simulink model "non_linear_model"  (R2018b)
settings: Solver=VariableStepAuto  StartTime=0.0  StopTime=10  RelTol=1e-3
values from neighbouring files (symbols this model uses):
  b = 1.5    [dettagli_auto.mat]
  ca = 1500    [dettagli_auto.mat]
  cp = 1600    [dettagli_auto.mat]
  g = 9.8    [dettagli_auto.mat]
  I = 24225    [dettagli_auto.mat]
  ka = 50000    [dettagli_auto.mat]
  Khinf = c2d(Khinf,Ts,'tustin')    [controllore_hinf.m]
  kp = 48000    [dettagli_auto.mat]
  lk = 1.125    [dettagli_auto.mat]
  m = 1600    [dettagli_auto.mat]
  noise_x = 0.0025    [dettagli_auto.mat]
  Ts = 0.01    [dettagli_auto.mat]
  x0 = [1.125 0 0 0]    [dettagli_auto.mat]
undefined symbols (not defined in the file or in its folder): int_lqg, int_pp, obs_lqg, obs_pp, sigbuilder_block
settings Model: Creator=cirom  LastModifiedBy=cirom

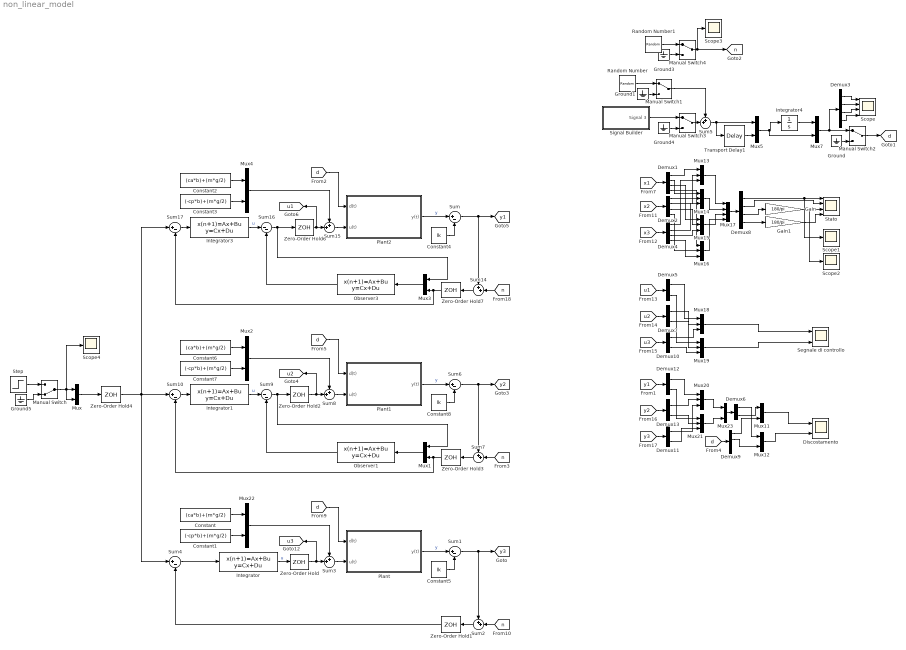
== system non_linear_model ==
  Constant : Constant  Value=(ca*b)+(m*g/2)
  Constant1 : Constant  Value=(-cp*b)+(m*g/2)
  Constant2 : Constant  Value=(ca*b)+(m*g/2)
  Constant3 : Constant  Value=(-cp*b)+(m*g/2)
  Constant4 : Constant  Value=lk
  Constant5 : Constant  Value=lk
  Constant6 : Constant  Value=(ca*b)+(m*g/2)
  Constant7 : Constant  Value=(-cp*b)+(m*g/2)
  Constant8 : Constant  Value=lk
  Demux{1..4,8..9} (6 alike) : Demux
  Demux{5..7,10..13} (7 alike) : Demux  Outputs=2
  Discostamento : Scope  NumInputPorts=2
  Gain : Gain  Gain=180/pi
  Gain1 : Gain  Gain=180/pi
  Ground{,1,3..5} (5 alike) : Ground
  Integrator : DiscreteStateSpace  A=Khinf.A  B=Khinf.B  C=Khinf.C  D=Khinf.D  SampleTime=-1
  Integrator1 : DiscreteStateSpace  A=int_lqg.A  B=int_lqg.B  C=int_lqg.C  D=int_lqg.D  SampleTime=-1
  Integrator3 : DiscreteStateSpace  A=int_pp.A  B=int_pp.B  C=int_pp.C  D=int_pp.D  SampleTime=-1
  Integrator4 : Integrator
  Manual Switch : ManualSwitch  CurrentSetting=0
  Manual Switch{1..4} (4 alike) : ManualSwitch
  Mux{,1..5,7,11..12,22..23} (11 alike) : Mux  Inputs=2
  Mux{13..16,18..21} (8 alike) : Mux  Inputs=3
  Mux17 : Mux
  Observer1 : DiscreteStateSpace  A=obs_lqg.A  B=obs_lqg.B  C=obs_lqg.C  D=obs_lqg.D  SampleTime=-1
  Observer3 : DiscreteStateSpace  A=obs_pp.A  B=obs_pp.B  C=obs_pp.C  D=obs_pp.D  SampleTime=-1
  Plant : Subsystem
  Plant1 : Subsystem
  Plant2 : Subsystem
  Random Number : RandomNumber  Variance=noise_x  SampleTime=0.01
  Random Number1 : RandomNumber  Variance=[1, 1] * 10^-4  SampleTime=0.001
  Scope : Scope  NumInputPorts=4
  Scope{1..4} (4 alike) : Scope
  Segnale di controllo : Scope  NumInputPorts=2
  Signal Builder : Subsystem  Tag=STV Subsys  LoadFcn=sigbuilder_block('load');  StartFcn=sigbuilder_block('start');  StopFcn=sigbuilder_block('stop');  ClipboardFcn=sigbuilder_block('clipboard');  mask(Sigbuilder block){tuvar=[0:10]}
      mask help: Simulink:masks:SigbuilderBlock_MD
      mask init:
      | if ~strcmp(get_param(bdroot(gcbh),'SimulationStatus'),'stopped') tuvar = sigbuilder_block('maskInit'); end
      settings: CopyFcn=sigbuilder_block('copy');  DeleteFcn=sigbuilder_block('delete');  ModelCloseFcn=sigbuilder_block('modelClose');  PreSaveFcn=sigbuilder_block('preSave');  PauseFcn=sigbuilder_block('pause');  ContinueFcn=sigbuilder_block('continue');  NameChangeFcn=sigbuilder_block('namechange');  OpenFcn=sigbuilder_block('open',[6 22.5 1012.5 455.25 ]);  CloseFcn=sigbuilder_block('close');
      mask Display: plot(0, 0, 100, 100,[2, 2, 32, 32, 2], [68, 8, 8, 68, 68],[32, 2], [38, 38], [32, 19, 2],[53, 60, 44], [32, 17, 17, 2],[16, 16, 31, 31]);txt = getActiveGroup(gcbh);text(2, 100, txt,'verticalAlignment', 'top');
  Stato : Scope  NumInputPorts=4
  Step : Step  After=0.05  SampleTime=0
  Sum{,1,4,6,10,17} (6 alike) : Sum  Inputs=|+-
  Sum{2..3,5,7..8,14..15} (7 alike) : Sum  Inputs=++|
  Sum16 : Sum  Inputs=|--
  Sum9 : Sum  Inputs=|--
  Transport Delay1 : TransportDelay  DelayTime=0.4
  Zero-Order Hold{,1..4,6..7} (7 alike) : ZeroOrderHold  SampleTime=Ts
  tag scope: d=global, n=global, u1=global, u2=global, u3=global, y1=global, y2=global, y3=global
  wires:
  Mux11/1 -> Discostamento/1
  [d] -> Demux9/1
  Mux17/1 -> Demux8/1
  Demux9/1 -> Mux11/2
  Demux9/2 -> Mux12/2
  Demux8/2 -> Stato/2
  Demux8/4 -> Gain1/1
  Gain1/1 -> Stato/4
  Demux8/1 -> Scope1/1, Stato/1
  Demux8/3 -> Gain/1
  Gain/1 -> Scope2/1, Stato/3
  Mux18/1 -> Segnale di controllo/1
  Mux19/1 -> Segnale di controllo/2
  [x2] -> Demux2/1
  [x3] -> Demux4/1
  Mux13/1 -> Mux17/1
  Mux14/1 -> Mux17/2
  Mux15/1 -> Mux17/3
  Mux16/1 -> Mux17/4
  Demux1/1 -> Mux13/1
  Demux2/1 -> Mux13/2
  Demux4/1 -> Mux13/3
  Demux1/2 -> Mux14/1
  Demux2/2 -> Mux14/2
  Demux4/2 -> Mux14/3
  Demux1/3 -> Mux15/1
  Demux2/3 -> Mux15/2
  Demux4/3 -> Mux15/3
  Demux1/4 -> Mux16/1
  Demux2/4 -> Mux16/2
  Demux4/4 -> Mux16/3
  Demux5/1 -> Mux18/1
  Demux5/2 -> Mux19/1
  Demux7/1 -> Mux18/2
  Demux7/2 -> Mux19/2
  Demux10/1 -> Mux18/3
  Demux10/2 -> Mux19/3
  [u2] -> Demux7/1
  [u3] -> Demux10/1
  Demux11/2 -> Mux21/3
  Demux12/2 -> Mux21/1
  Demux12/1 -> Mux20/1
  Mux20/1 -> Mux23/1
  Demux13/2 -> Mux21/2
  Mux23/1 -> Demux6/1
  Demux13/1 -> Mux20/2
  Demux11/1 -> Mux20/3
  Mux21/1 -> Mux23/2
  [y2] -> Demux13/1
  [y3] -> Demux11/1
  Manual Switch4/1 -> Scope3/1, [n]
  Ground3/1 -> Manual Switch4/2
  Random Number1/1 -> Manual Switch4/1
  Demux6/1 -> Mux12/1
  Demux6/2 -> Mux11/1
  Integrator3/1 -> Sum16/1  "u"
  [d] -> Plant2/1(d(t))
  Plant2/1(y(t)) -> Sum/1  "y"
  Sum17/1 -> Integrator3/1
  Mux3/1 -> Observer3/1
  Constant2/1 -> Mux4/1
  Observer3/1 -> Sum16/2
  Sum15/1 -> Plant2/2(u(t))
  Mux4/1 -> Sum15/1
  [n] -> Sum14/2
  Constant3/1 -> Mux4/2
  Zero-Order Hold7/1 -> Sum17/2, Mux3/2
  Sum16/1 -> Mux3/1, Zero-Order Hold6/1
  Sum14/1 -> Zero-Order Hold7/1
  Sum/1 -> Sum14/1, [y1]
  Zero-Order Hold6/1 -> [u1], Sum15/2
  Constant4/1 -> Sum/2
  Demux3/4 -> Scope/4
  Demux3/3 -> Scope/3
  Random Number/1 -> Manual Switch1/1
  Ground4/1 -> Manual Switch3/2
  Demux3/2 -> Scope/2
  Mux7/1 -> Demux3/1, Manual Switch2/1
  Manual Switch3/1 -> Sum5/2
  Ground/1 -> Manual Switch2/2
  Ground1/1 -> Manual Switch1/2
  Manual Switch1/1 -> Sum5/1
  Sum5/1 -> Transport Delay1/1, Mux5/1
  Manual Switch2/1 -> [d]
  Mux5/1 -> Mux7/2, Integrator4/1
  Transport Delay1/1 -> Mux5/2
  Demux3/1 -> Scope/1
  Integrator4/1 -> Mux7/1
  Signal Builder/1(Signal 3) -> Manual Switch3/1
  [x1] -> Demux1/1
  [u1] -> Demux5/1
  [y1] -> Demux12/1
  Sum3/1 -> Plant/2(u(t))
  Zero-Order Hold/1 -> Sum3/2, [u3]
  [n] -> Sum2/2
  Plant/1(y(t)) -> Sum1/1  "y"
  Constant5/1 -> Sum1/2
  Sum2/1 -> Zero-Order Hold1/1
  Integrator/1 -> Zero-Order Hold/1  "u"
  [d] -> Plant/1(d(t))
  Mux22/1 -> Sum3/1
  Zero-Order Hold4/1 -> Sum4/1, Sum17/1, Sum10/1
  Constant1/1 -> Mux22/2
  Sum1/1 -> Sum2/1, [y3]
  Zero-Order Hold1/1 -> Sum4/2
  Sum4/1 -> Integrator/1
  Constant/1 -> Mux22/1
  Mux12/1 -> Discostamento/2
  [n] -> Sum7/2
  Zero-Order Hold2/1 -> [u2], Sum8/2
  Sum9/1 -> Mux1/1, Zero-Order Hold2/1
  Mux1/1 -> Observer1/1
  Observer1/1 -> Sum9/2
  Sum6/1 -> Sum7/1, [y2]
  Sum7/1 -> Zero-Order Hold3/1
  Integrator1/1 -> Sum9/1  "u"
  Constant7/1 -> Mux2/2
  Mux2/1 -> Sum8/1
  Sum8/1 -> Plant1/2(u(t))
  Sum10/1 -> Integrator1/1
  Plant1/1(y(t)) -> Sum6/1  "y"
  [d] -> Plant1/1(d(t))
  Constant6/1 -> Mux2/1
  Zero-Order Hold3/1 -> Sum10/2, Mux1/2
  Constant8/1 -> Sum6/2
  Step/1 -> Manual Switch/1
  Ground5/1 -> Manual Switch/2
  Manual Switch/1 -> Scope4/1, Mux/2, Mux/1
  Mux/1 -> Zero-Order Hold4/1

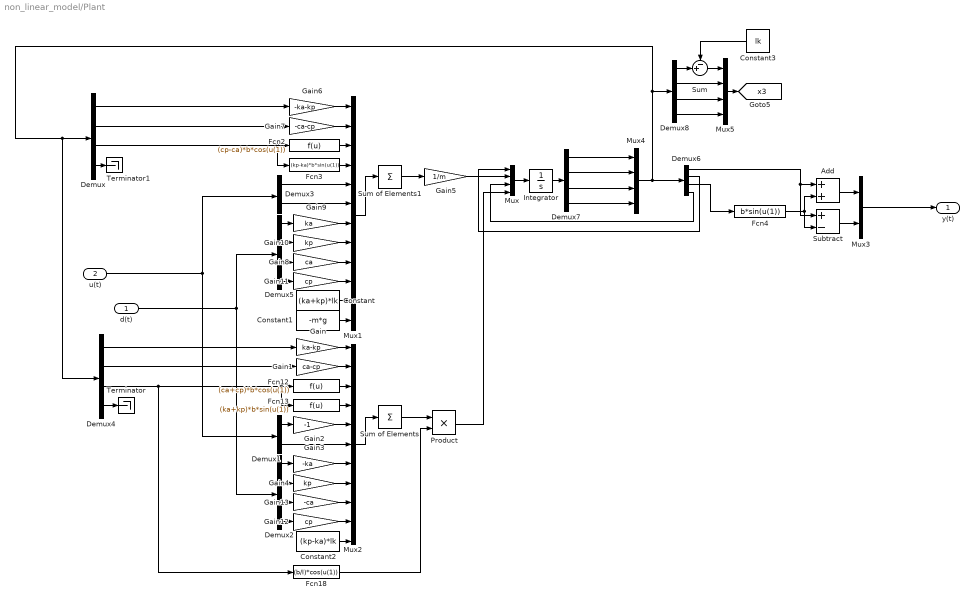
== system non_linear_model/Plant ==
  d(t) : Inport
  u(t) : Inport  Port=2
  Add : Sum
  Constant : Constant  Value=(ka+kp)*lk
  Constant1 : Constant  Value=-m*g
  Constant2 : Constant  Value=(kp-ka)*lk
  Constant3 : Constant  Value=lk
  Demux{,2,4..8} (7 alike) : Demux
  Demux1 : Demux  Outputs=2
  Demux3 : Demux  Outputs=2
  Fcn12 : Fcn  Expr=(ca+cp)*b*cos(u(1))
  Fcn13 : Fcn  Expr=(ka+kp)*b*sin(u(1))
  Fcn18 : Fcn  Expr=(b/I)*cos(u(1))
  Fcn2 : Fcn  Expr=(cp-ca)*b*cos(u(1))
  Fcn3 : Fcn  Expr=(kp-ka)*b*sin(u(1))
  Fcn4 : Fcn  Expr=b*sin(u(1))
  Gain : Gain  Gain=ka-kp
  Gain1 : Gain  Gain=ca-cp
  Gain10 : Gain  Gain=kp
  Gain11 : Gain  Gain=cp
  Gain12 : Gain  Gain=cp
  Gain13 : Gain  Gain=-ca
  Gain2 : Gain  Gain=-1
  Gain3 : Gain  Gain=-ka
  Gain4 : Gain  Gain=kp
  Gain5 : Gain  Gain=1/m
  Gain6 : Gain  Gain=-ka-kp
  Gain7 : Gain  Gain=-ca-cp
  Gain8 : Gain  Gain=ca
  Gain9 : Gain  Gain=ka
  Integrator : Integrator  InitialCondition=x0
  Mux : Mux
  Mux1 : Mux  Inputs=12
  Mux2 : Mux  Inputs=11
  Mux3 : Mux  Inputs=2
  Mux4 : Mux
  Mux5 : Mux
  Product : Product
  Subtract : Sum  Inputs=+-
  Sum : Sum  Inputs=-+|
  Sum of Elements : Sum  Inputs=+
  Sum of Elements1 : Sum  Inputs=+
  Terminator : Terminator
  Terminator1 : Terminator
  y(t) : Outport
  tag scope: x3=global
  wires:
  Mux/1 -> Integrator/1
  u(t)/1 -> Demux3/1, Demux1/1
  Mux1/1 -> Sum of Elements1/1
  Demux2/1 -> Gain3/1
  Demux2/2 -> Gain4/1
  Gain3/1 -> Mux2/7
  Gain4/1 -> Mux2/8
  Gain/1 -> Mux2/1
  Gain1/1 -> Mux2/2
  Fcn12/1 -> Mux2/3
  Mux2/1 -> Sum of Elements/1
  Fcn13/1 -> Mux2/4
  Sum of Elements/1 -> Product/1
  Fcn18/1 -> Product/2
  Gain2/1 -> Mux2/5
  Product/1 -> Mux/4
  Sum of Elements1/1 -> Gain5/1
  Gain5/1 -> Mux/2
  Gain9/1 -> Mux1/7
  Demux3/1 -> Mux1/5
  Fcn2/1 -> Mux1/3
  Gain10/1 -> Mux1/8
  Fcn3/1 -> Mux1/4
  Gain7/1 -> Mux1/2
  Gain6/1 -> Mux1/1
  Demux3/2 -> Mux1/6
  Demux1/1 -> Gain2/1
  Demux1/2 -> Mux2/6
  d(t)/1 -> Demux2/1, Demux5/1
  Demux/1 -> Gain6/1
  Demux/2 -> Gain7/1
  Demux/3 -> Fcn3/1, Fcn2/1
  Demux4/1 -> Gain/1
  Demux4/2 -> Gain1/1
  Demux4/3 -> Fcn18/1, Fcn13/1, Fcn12/1
  Demux4/4 -> Terminator/1
  Demux5/1 -> Gain9/1
  Demux5/2 -> Gain10/1
  Demux/4 -> Terminator1/1
  Demux6/2 -> Mux/1
  Demux6/4 -> Mux/3
  Demux6/1 -> Subtract/1, Add/1
  Fcn4/1 -> Add/2, Subtract/2
  Add/1 -> Mux3/1
  Subtract/1 -> Mux3/2
  Mux3/1 -> y(t)/1
  Demux6/3 -> Fcn4/1
  Mux4/1 -> Demux8/1, Demux4/1, Demux/1, Demux6/1
  Integrator/1 -> Demux7/1
  Demux7/1 -> Mux4/1
  Demux7/2 -> Mux4/2
  Demux7/3 -> Mux4/3
  Demux7/4 -> Mux4/4
  Demux5/3 -> Gain8/1
  Demux5/4 -> Gain11/1
  Gain8/1 -> Mux1/9
  Gain11/1 -> Mux1/10
  Demux2/3 -> Gain13/1
  Demux2/4 -> Gain12/1
  Gain13/1 -> Mux2/9
  Gain12/1 -> Mux2/10
  Constant/1 -> Mux1/11
  Constant1/1 -> Mux1/12
  Constant2/1 -> Mux2/11
  Sum/1 -> Mux5/1
  Demux8/1 -> Sum/2
  Demux8/2 -> Mux5/2
  Demux8/3 -> Mux5/3
  Demux8/4 -> Mux5/4
  Mux5/1 -> [x3]
  Constant3/1 -> Sum/1

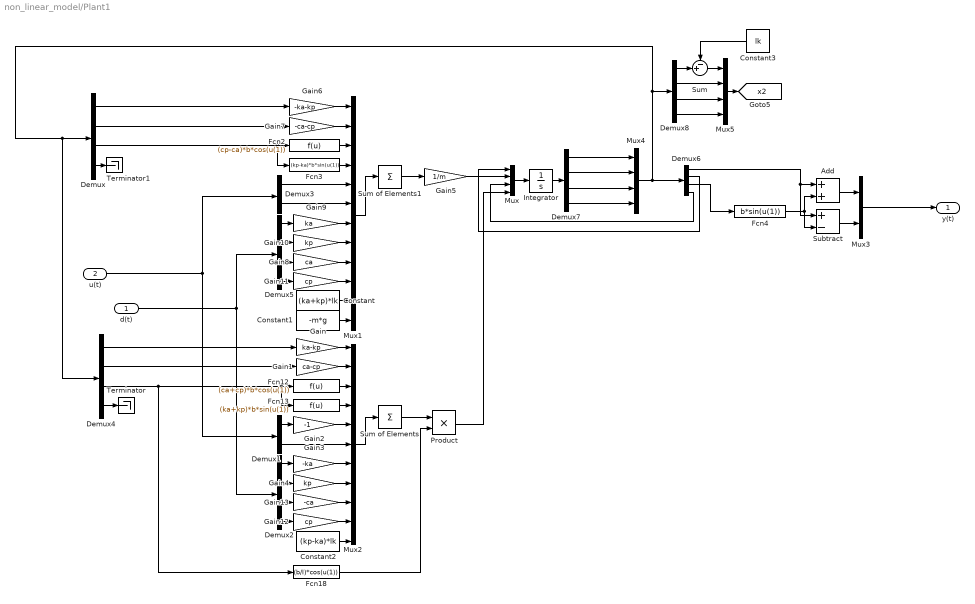
== system non_linear_model/Plant1 ==
  d(t) : Inport
  u(t) : Inport  Port=2
  Add : Sum
  Constant : Constant  Value=(ka+kp)*lk
  Constant1 : Constant  Value=-m*g
  Constant2 : Constant  Value=(kp-ka)*lk
  Constant3 : Constant  Value=lk
  Demux{,2,4..8} (7 alike) : Demux
  Demux1 : Demux  Outputs=2
  Demux3 : Demux  Outputs=2
  Fcn12 : Fcn  Expr=(ca+cp)*b*cos(u(1))
  Fcn13 : Fcn  Expr=(ka+kp)*b*sin(u(1))
  Fcn18 : Fcn  Expr=(b/I)*cos(u(1))
  Fcn2 : Fcn  Expr=(cp-ca)*b*cos(u(1))
  Fcn3 : Fcn  Expr=(kp-ka)*b*sin(u(1))
  Fcn4 : Fcn  Expr=b*sin(u(1))
  Gain : Gain  Gain=ka-kp
  Gain1 : Gain  Gain=ca-cp
  Gain10 : Gain  Gain=kp
  Gain11 : Gain  Gain=cp
  Gain12 : Gain  Gain=cp
  Gain13 : Gain  Gain=-ca
  Gain2 : Gain  Gain=-1
  Gain3 : Gain  Gain=-ka
  Gain4 : Gain  Gain=kp
  Gain5 : Gain  Gain=1/m
  Gain6 : Gain  Gain=-ka-kp
  Gain7 : Gain  Gain=-ca-cp
  Gain8 : Gain  Gain=ca
  Gain9 : Gain  Gain=ka
  Integrator : Integrator  InitialCondition=x0
  Mux : Mux
  Mux1 : Mux  Inputs=12
  Mux2 : Mux  Inputs=11
  Mux3 : Mux  Inputs=2
  Mux4 : Mux
  Mux5 : Mux
  Product : Product
  Subtract : Sum  Inputs=+-
  Sum : Sum  Inputs=-+|
  Sum of Elements : Sum  Inputs=+
  Sum of Elements1 : Sum  Inputs=+
  Terminator : Terminator
  Terminator1 : Terminator
  y(t) : Outport
  tag scope: x2=global
  wires:
  Mux/1 -> Integrator/1
  u(t)/1 -> Demux3/1, Demux1/1
  Mux1/1 -> Sum of Elements1/1
  Demux2/1 -> Gain3/1
  Demux2/2 -> Gain4/1
  Gain3/1 -> Mux2/7
  Gain4/1 -> Mux2/8
  Gain/1 -> Mux2/1
  Gain1/1 -> Mux2/2
  Fcn12/1 -> Mux2/3
  Mux2/1 -> Sum of Elements/1
  Fcn13/1 -> Mux2/4
  Sum of Elements/1 -> Product/1
  Fcn18/1 -> Product/2
  Gain2/1 -> Mux2/5
  Product/1 -> Mux/4
  Sum of Elements1/1 -> Gain5/1
  Gain5/1 -> Mux/2
  Gain9/1 -> Mux1/7
  Demux3/1 -> Mux1/5
  Fcn2/1 -> Mux1/3
  Gain10/1 -> Mux1/8
  Fcn3/1 -> Mux1/4
  Gain7/1 -> Mux1/2
  Gain6/1 -> Mux1/1
  Demux3/2 -> Mux1/6
  Demux1/1 -> Gain2/1
  Demux1/2 -> Mux2/6
  d(t)/1 -> Demux2/1, Demux5/1
  Demux/1 -> Gain6/1
  Demux/2 -> Gain7/1
  Demux/3 -> Fcn3/1, Fcn2/1
  Demux4/1 -> Gain/1
  Demux4/2 -> Gain1/1
  Demux4/3 -> Fcn18/1, Fcn13/1, Fcn12/1
  Demux4/4 -> Terminator/1
  Demux5/1 -> Gain9/1
  Demux5/2 -> Gain10/1
  Demux/4 -> Terminator1/1
  Demux6/2 -> Mux/1
  Demux6/4 -> Mux/3
  Demux6/1 -> Subtract/1, Add/1
  Fcn4/1 -> Add/2, Subtract/2
  Add/1 -> Mux3/1
  Subtract/1 -> Mux3/2
  Mux3/1 -> y(t)/1
  Demux6/3 -> Fcn4/1
  Mux4/1 -> Demux8/1, Demux4/1, Demux/1, Demux6/1
  Integrator/1 -> Demux7/1
  Demux7/1 -> Mux4/1
  Demux7/2 -> Mux4/2
  Demux7/3 -> Mux4/3
  Demux7/4 -> Mux4/4
  Demux5/3 -> Gain8/1
  Demux5/4 -> Gain11/1
  Gain8/1 -> Mux1/9
  Gain11/1 -> Mux1/10
  Demux2/3 -> Gain13/1
  Demux2/4 -> Gain12/1
  Gain13/1 -> Mux2/9
  Gain12/1 -> Mux2/10
  Constant/1 -> Mux1/11
  Constant1/1 -> Mux1/12
  Constant2/1 -> Mux2/11
  Sum/1 -> Mux5/1
  Demux8/1 -> Sum/2
  Demux8/2 -> Mux5/2
  Demux8/3 -> Mux5/3
  Demux8/4 -> Mux5/4
  Mux5/1 -> [x2]
  Constant3/1 -> Sum/1

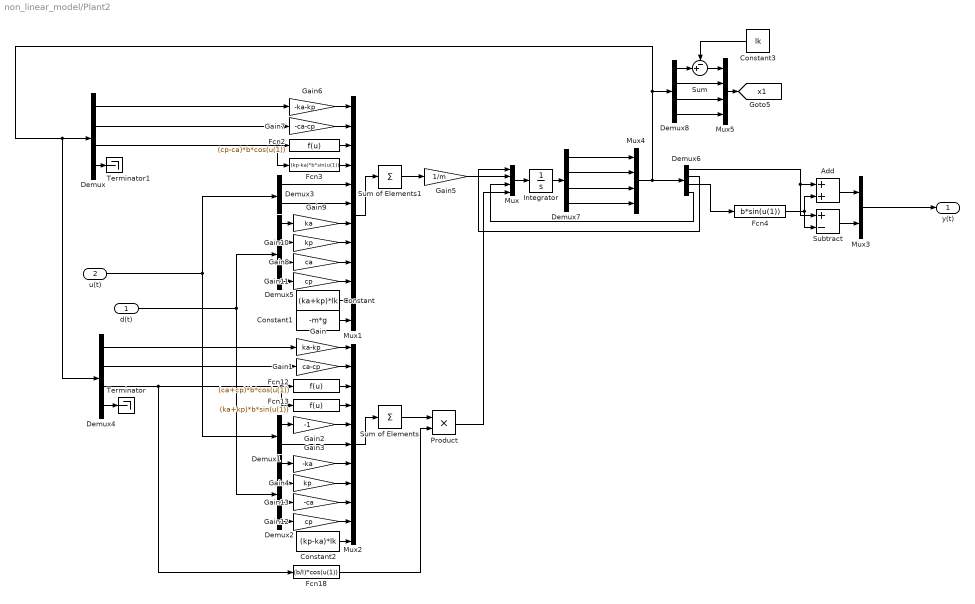
== system non_linear_model/Plant2 ==
  d(t) : Inport
  u(t) : Inport  Port=2
  Add : Sum
  Constant : Constant  Value=(ka+kp)*lk
  Constant1 : Constant  Value=-m*g
  Constant2 : Constant  Value=(kp-ka)*lk
  Constant3 : Constant  Value=lk
  Demux{,2,4..8} (7 alike) : Demux
  Demux1 : Demux  Outputs=2
  Demux3 : Demux  Outputs=2
  Fcn12 : Fcn  Expr=(ca+cp)*b*cos(u(1))
  Fcn13 : Fcn  Expr=(ka+kp)*b*sin(u(1))
  Fcn18 : Fcn  Expr=(b/I)*cos(u(1))
  Fcn2 : Fcn  Expr=(cp-ca)*b*cos(u(1))
  Fcn3 : Fcn  Expr=(kp-ka)*b*sin(u(1))
  Fcn4 : Fcn  Expr=b*sin(u(1))
  Gain : Gain  Gain=ka-kp
  Gain1 : Gain  Gain=ca-cp
  Gain10 : Gain  Gain=kp
  Gain11 : Gain  Gain=cp
  Gain12 : Gain  Gain=cp
  Gain13 : Gain  Gain=-ca
  Gain2 : Gain  Gain=-1
  Gain3 : Gain  Gain=-ka
  Gain4 : Gain  Gain=kp
  Gain5 : Gain  Gain=1/m
  Gain6 : Gain  Gain=-ka-kp
  Gain7 : Gain  Gain=-ca-cp
  Gain8 : Gain  Gain=ca
  Gain9 : Gain  Gain=ka
  Integrator : Integrator  InitialCondition=x0
  Mux : Mux
  Mux1 : Mux  Inputs=12
  Mux2 : Mux  Inputs=11
  Mux3 : Mux  Inputs=2
  Mux4 : Mux
  Mux5 : Mux
  Product : Product
  Subtract : Sum  Inputs=+-
  Sum : Sum  Inputs=-+|
  Sum of Elements : Sum  Inputs=+
  Sum of Elements1 : Sum  Inputs=+
  Terminator : Terminator
  Terminator1 : Terminator
  y(t) : Outport
  tag scope: x1=global
  wires:
  Mux/1 -> Integrator/1
  u(t)/1 -> Demux3/1, Demux1/1
  Mux1/1 -> Sum of Elements1/1
  Demux2/1 -> Gain3/1
  Demux2/2 -> Gain4/1
  Gain3/1 -> Mux2/7
  Gain4/1 -> Mux2/8
  Gain/1 -> Mux2/1
  Gain1/1 -> Mux2/2
  Fcn12/1 -> Mux2/3
  Mux2/1 -> Sum of Elements/1
  Fcn13/1 -> Mux2/4
  Sum of Elements/1 -> Product/1
  Fcn18/1 -> Product/2
  Gain2/1 -> Mux2/5
  Product/1 -> Mux/4
  Sum of Elements1/1 -> Gain5/1
  Gain5/1 -> Mux/2
  Gain9/1 -> Mux1/7
  Demux3/1 -> Mux1/5
  Fcn2/1 -> Mux1/3
  Gain10/1 -> Mux1/8
  Fcn3/1 -> Mux1/4
  Gain7/1 -> Mux1/2
  Gain6/1 -> Mux1/1
  Demux3/2 -> Mux1/6
  Demux1/1 -> Gain2/1
  Demux1/2 -> Mux2/6
  d(t)/1 -> Demux2/1, Demux5/1
  Demux/1 -> Gain6/1
  Demux/2 -> Gain7/1
  Demux/3 -> Fcn3/1, Fcn2/1
  Demux4/1 -> Gain/1
  Demux4/2 -> Gain1/1
  Demux4/3 -> Fcn18/1, Fcn13/1, Fcn12/1
  Demux4/4 -> Terminator/1
  Demux5/1 -> Gain9/1
  Demux5/2 -> Gain10/1
  Demux/4 -> Terminator1/1
  Demux6/2 -> Mux/1
  Demux6/4 -> Mux/3
  Demux6/1 -> Subtract/1, Add/1
  Fcn4/1 -> Add/2, Subtract/2
  Add/1 -> Mux3/1
  Subtract/1 -> Mux3/2
  Mux3/1 -> y(t)/1
  Demux6/3 -> Fcn4/1
  Mux4/1 -> Demux8/1, Demux4/1, Demux/1, Demux6/1
  Integrator/1 -> Demux7/1
  Demux7/1 -> Mux4/1
  Demux7/2 -> Mux4/2
  Demux7/3 -> Mux4/3
  Demux7/4 -> Mux4/4
  Demux5/3 -> Gain8/1
  Demux5/4 -> Gain11/1
  Gain8/1 -> Mux1/9
  Gain11/1 -> Mux1/10
  Demux2/3 -> Gain13/1
  Demux2/4 -> Gain12/1
  Gain13/1 -> Mux2/9
  Gain12/1 -> Mux2/10
  Constant/1 -> Mux1/11
  Constant1/1 -> Mux1/12
  Constant2/1 -> Mux2/11
  Sum/1 -> Mux5/1
  Demux8/1 -> Sum/2
  Demux8/2 -> Mux5/2
  Demux8/3 -> Mux5/3
  Demux8/4 -> Mux5/4
  Mux5/1 -> [x1]
  Constant3/1 -> Sum/1

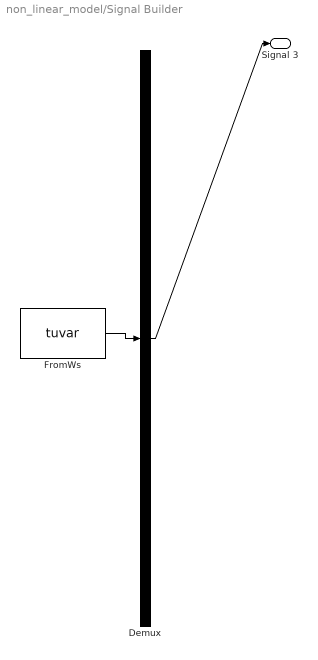
== system non_linear_model/Signal Builder ==
  Demux : Demux  Tag=STV Demux  Outputs=1
  FromWs : FromWorkspace  Tag=STV FromWs  VariableName=tuvar  SampleTime=0
      SigBuilderData=|
      | common.afterFinalStr = 'Extrapolate'
      | common.sampleTime = 0
      | dataSet.timeRange = [0 10]
      | dataSet.name = 'Group 1'
      | sbobj.Groups.Name = 'Group 1'
      | sbobj.Groups.Signals.Name = 'Signal 3'
      | sbobj.Groups.Signals.XData = [0 0.4 0.8 1.6 2 2.4 10]
      | sbobj.Groups.Signals.YData = [0 0.1 0.1 -0.1 -0.1 0 0]
  Signal 3 : Outport  Tag=STV Outport
  wires:
  FromWs/1 -> Demux/1
  Demux/1 -> Signal 3/1
